simulink model "UC613"  (R2022b)
settings: Solver=VariableStepAuto  StartTime=0.0  StopTime=10.0  RelTol=1e-3
settings Model: DataDictionary=Optimate_PhysicalArchiDD.sldd  Creator=TO41629  LastModifiedBy=TO41629

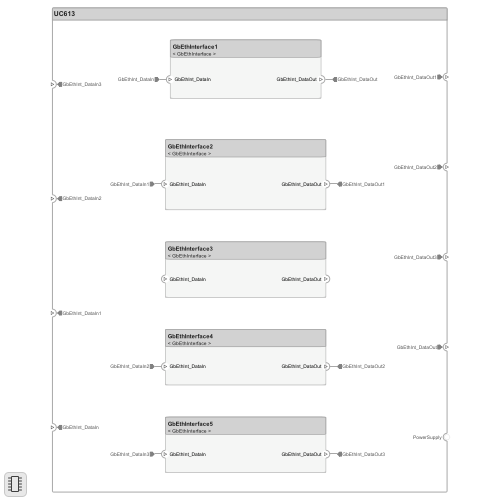
[thumbnail: Simulink's stored preview of the top-level diagram]
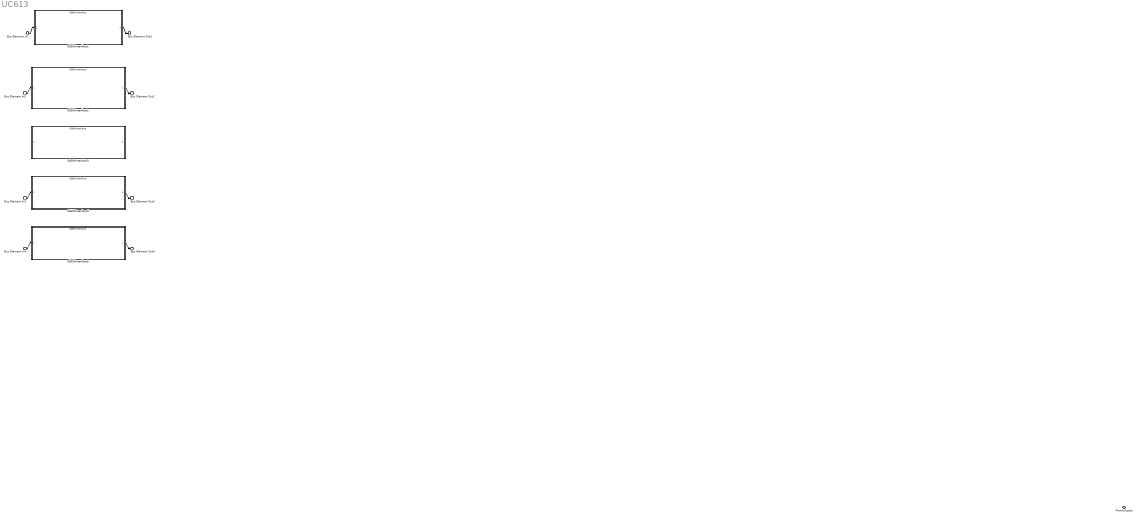
== system UC613 ==
  Bus Element In4 : Inport  PortName=GbEthInt_DataIn3
  Bus Element In3 : Inport  Port=2  PortName=GbEthInt_DataIn2
  Bus Element In2 : Inport  Port=3  PortName=GbEthInt_DataIn1
  Bus Element In1 : Inport  Port=4  PortName=GbEthInt_DataIn
  GbEthInterface{1..5} (5 alike) : ModelReference  ModelNameDialog=GbEthInterface  UsingDefaultArgumentValue=0,0,0  SimulationMode=Normal  ModelReferenceVersion=1.27
      settings: PortSchema="{\"entries\":[{\"content\":{\"headerSize\":38,\"margin\":15,\"minimumSpacing\":25,\"sides\":[{\"content\":{\"connectorIds\":[\"In1\"]},\"type\":\"ConnectorPlacement.EquallySpacedRectSide\",\"uuid\":\"1de95e92-70ae-43a9-bde0-2190bb61790d\"},{\"content\":{\"connectorIds\":[\"Out1\"],\"side\":\"RIGHT\"},\"type\":\"ConnectorPlacement.EquallySpacedRectSide\",\"uuid\":\"1b5d6d3c-e0d8-4f64-8598-70a2a995425a\"},{\"content\":{\"connectorIds\":[],\"side\":\"TOP\"},\"type\":\"ConnectorPlacement.EquallySpacedRectSide\",\"uuid\":\"7db0e0c1-3793-4c9b-91c6-efc6298ad516\"}]},\"type\":\"ConnectorPlacement.EquallySpacedConnector\",\"uuid\":\"f8322e21-ae52-44ed-a1f2-cf6a6dc8b30a\"}],\"packageUris\":[\"http://schema.mathworks.com/mf0/Connector/R2020b\"],\"version\":\"1.0\"}"
  PowerSupply : PMIOPort  Side=Right
  Bus Element Out2 : Outport  PortName=GbEthInt_DataOut1
  Bus Element Out3 : Outport  Port=2  PortName=GbEthInt_DataOut2
  Bus Element Out4 : Outport  Port=3  PortName=GbEthInt_DataOut3
  Bus Element Out1 : Outport  Port=4  PortName=GbEthInt_DataOut
  wires:
  GbEthInterface1/1 -> Bus Element Out1/1
  Bus Element In1/1 -> GbEthInterface1/1
  Bus Element In2/1 -> GbEthInterface2/1
  GbEthInterface2/1 -> Bus Element Out2/1
  Bus Element In3/1 -> GbEthInterface4/1
  GbEthInterface4/1 -> Bus Element Out3/1
  Bus Element In4/1 -> GbEthInterface5/1
  GbEthInterface5/1 -> Bus Element Out4/1
